simulink model "TOC_simulation"  (R2018a)
settings: Solver=VariableStepAuto  StartTime=0.0  StopTime=300  RelTol=1e-3
libraries: dspsigops x1
settings Model: Creator=stefan  LastModifiedBy=stefan

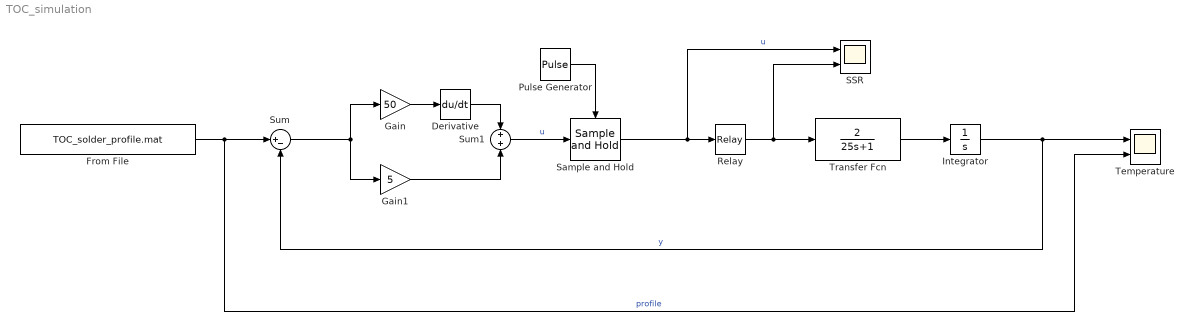
== system TOC_simulation ==
  Derivative : Derivative
  From File : FromFile  FileName=TOC_solder_profile.mat  SampleTime=0
  Gain : Gain  Gain=50
  Gain1 : Gain  Gain=5
  Integrator : Integrator  InitialCondition=25
  Pulse Generator : DiscretePulseGenerator  PulseType=Time based  Period=0.5  PulseWidth=50
  Relay : Relay  OnSwitchValue=10  OffSwitchValue=5
  SSR : Scope  NumInputPorts=2
  Sample and Hold : dspsigops/Sample and Hold  trig=Rising edge  initCond=0  latchinput=off
  Sum : Sum  Inputs=|+-
  Sum1 : Sum
  Temperature : Scope  NumInputPorts=2
  Transfer Fcn : TransferFcn  Numerator=2  Denominator=[25 1]
  wires:
  From File/1 -> Sum/1, Temperature/2  "profile"
  Transfer Fcn/1 -> Integrator/1
  Sample and Hold/1 -> SSR/1, Relay/1  "u"
  Sum/1 -> Gain1/1, Gain/1
  Gain/1 -> Derivative/1
  Derivative/1 -> Sum1/1
  Gain1/1 -> Sum1/2
  Relay/1 -> SSR/2, Transfer Fcn/1
  Integrator/1 -> Temperature/1, Sum/2  "y"
  Sum1/1 -> Sample and Hold/1  "u"
  Pulse Generator/1 -> Sample and Hold/Trigger
